simulink model "test_model_2018a1"  (R2018a)
settings: Solver=VariableStepAuto  StartTime=0.0  StopTime=4  RelTol=1e-3
values from neighbouring files (symbols this model uses):
  A = sys_d.A    [discreteTest.m]    (also in discreteTestAttacked.m)
  B = sys_d.B    [discreteTest.m]    (also in discreteTestAttacked.m)
  C = sys_d.C    [discreteTest.m]    (also in discreteTestAttacked.m)
  delta = steeringAngle(i)*(pi/180)*steering_ratio    [discreteTest.m]    (also in discreteTestAttacked.m)
  K = [   5.261, -0.023 ... (first row only)    [discreteTest.m]    (also in discreteTestAttacked.m)
  Ts = 0.04    [discreteTest.m]    (also in discreteTestAttacked.m)
undefined symbols (not defined in the file or in its folder): canChannel, L
libraries: canlib x6, canmsglib x4
settings Model: Creator=Shreyash  LastModifiedBy=Shreyash
settings SolverCC: AlgebraicLoopSolver=LineSearch

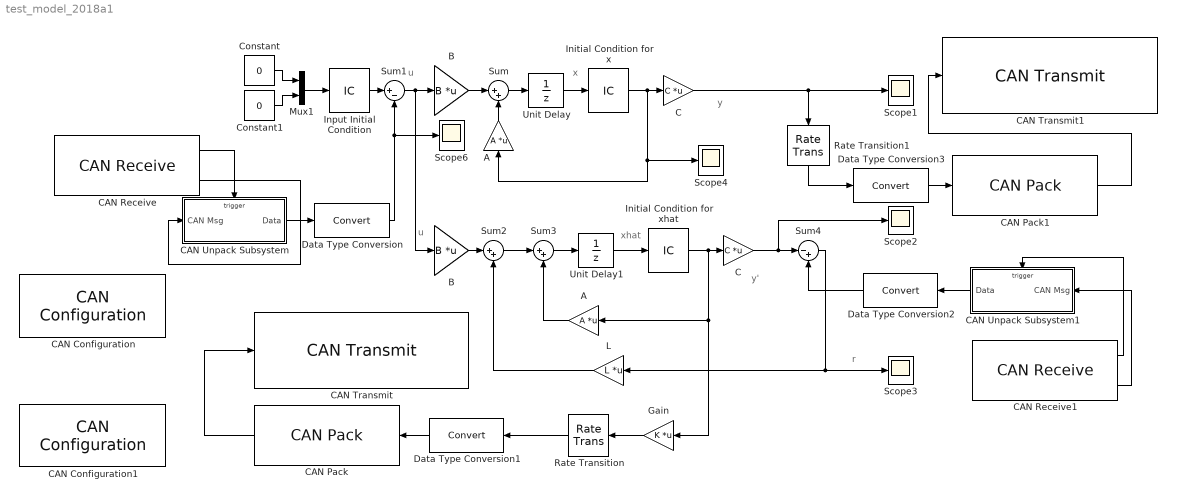
== system test_model_2018a1 ==
  note: y
  note: r
  note: y'
  note: u
  note: u
  note: x
  note: xhat
  A : Gain  Gain=A  Multiplication=Matrix(K*u)
  "A " : Gain  Gain=A  Multiplication=Matrix(K*u)
  B : Gain  Gain=B  Multiplication=Matrix(K*u)
  "B " : Gain  Gain=B  Multiplication=Matrix(K*u)
  C : Gain  Gain=C  Multiplication=Matrix(K*u)
  "C " : Gain  Gain=C  Multiplication=Matrix(K*u)
  CAN Configuration : canlib/CAN Configuration  BlockHandle=11.0004  DeviceMenu=MathWorks Virtual 1 (Channel 1)  Device=MathWorks Virtual 1 (Channel 1)  ObjConstructor=canChannel('MathWorks', 'Virtual 1', 1)  BusSpeed=500000  EnableBitParameters=off  AckMode=Normal
      settings: SourceProductName=Vehicle Network Toolbox  SourceProductBaseCode=VN
  CAN Configuration1 : canlib/CAN Configuration  BlockHandle=12.0004  DeviceMenu=MathWorks Virtual 1 (Channel 2)  Device=MathWorks Virtual 1 (Channel 2)  ObjConstructor=canChannel('MathWorks', 'Virtual 1', 2)  BusSpeed=500000  EnableBitParameters=off  AckMode=Normal
      settings: SourceProductName=Vehicle Network Toolbox  SourceProductBaseCode=VN
  CAN Pack : canmsglib/CAN Pack  MsgList=(none)  MsgName=CAN Msg  MsgIDType=Standard (11-bit identifier)  MsgIdentifier=500  MsgLength=8  NSignals=0  StartBits=0  SignalSizes=0  ByteOrders=0  DataTypes=0  MultiplexTypes=0  MultiplexValues=0  Factors=0  Offsets=0  Minimums=0  Maximums=0  Remote=off  ApplyMinMax=off  BusOutput=off
      settings: SourceProductName=Vehicle Network Toolbox  SourceProductBaseCode=VN  DataFormat=raw data
  CAN Pack1 : canmsglib/CAN Pack  MsgList=(none)  MsgName=CAN Msg  MsgIDType=Standard (11-bit identifier)  MsgIdentifier=500  MsgLength=8  NSignals=0  StartBits=0  SignalSizes=0  ByteOrders=0  DataTypes=0  MultiplexTypes=0  MultiplexValues=0  Factors=0  Offsets=0  Minimums=0  Maximums=0  Remote=off  ApplyMinMax=off  BusOutput=off
      settings: SourceProductName=Vehicle Network Toolbox  SourceProductBaseCode=VN  DataFormat=raw data
  CAN Receive : canlib/CAN Receive  BlockHandle=17.0004  DeviceMenu=MathWorks Virtual 1 (Channel 2)  Device=MathWorks Virtual 1 (Channel 2)  ObjConstructor=canChannel('MathWorks', 'Virtual 1', 2)  EnableStandardIDsFilter=off  StandardIDs=0  EnableExtendedIDsFilter=off  ExtendedIDs=0  SampleTime=0.04  MsgsPerTimestep=all  StdIDsCombo=Allow all  ExtIDsCombo=Allow all  InternalFilterUpdateStatus=on  BusOutput=off
      settings: SourceProductName=Vehicle Network Toolbox  SourceProductBaseCode=VN
  CAN Receive1 : canlib/CAN Receive  BlockHandle=18.0004  DeviceMenu=MathWorks Virtual 1 (Channel 2)  Device=MathWorks Virtual 1 (Channel 2)  ObjConstructor=canChannel('MathWorks', 'Virtual 1', 2)  EnableStandardIDsFilter=off  StandardIDs=0  EnableExtendedIDsFilter=off  ExtendedIDs=0  SampleTime=0.04  MsgsPerTimestep=all  StdIDsCombo=Allow all  ExtIDsCombo=Allow all  InternalFilterUpdateStatus=on  BusOutput=off
      settings: SourceProductName=Vehicle Network Toolbox  SourceProductBaseCode=VN
  CAN Transmit : canlib/CAN Transmit  BlockHandle=19.0004  DeviceMenu=MathWorks Virtual 1 (Channel 1)  Device=MathWorks Virtual 1 (Channel 1)  ObjConstructor=canChannel('MathWorks', 'Virtual 1', 1)  EnablePeriodicTransmit=on  MessagePeriod=0.04
      settings: SourceProductName=Vehicle Network Toolbox  SourceProductBaseCode=VN
  CAN Transmit1 : canlib/CAN Transmit  BlockHandle=20.0004  DeviceMenu=MathWorks Virtual 1 (Channel 1)  Device=MathWorks Virtual 1 (Channel 1)  ObjConstructor=canChannel('MathWorks', 'Virtual 1', 1)  EnablePeriodicTransmit=on  MessagePeriod=0.04
      settings: SourceProductName=Vehicle Network Toolbox  SourceProductBaseCode=VN
  CAN Unpack Subsystem : Subsystem  TreatAsAtomicUnit=on
  CAN Unpack Subsystem1 : Subsystem  TreatAsAtomicUnit=on
  Constant : Constant  Value=0
  Constant1 : Constant  Value=0
  Data Type Conversion : DataTypeConversion  SaturateOnIntegerOverflow=on
  Data Type Conversion1 : DataTypeConversion
  Data Type Conversion2 : DataTypeConversion  SaturateOnIntegerOverflow=on
  Data Type Conversion3 : DataTypeConversion
  Gain : Gain  Gain=K  Multiplication=Matrix(K*u)
  Initial Condition for x : InitialCondition  Value=[0.0005062279;0.0162158827]
  Initial Condition for xhat : InitialCondition  Value=[0;0]
  Input Initial Condition : InitialCondition  Value=[delta;0]
  L : Gain  Gain=L  Multiplication=Matrix(K*u)
  Mux1 : Mux  Inputs=2
  Rate Transition : RateTransition  Deterministic=off  InitialCondition=Ts  OutPortSampleTime=Ts
  Rate Transition1 : RateTransition  InitialCondition=Ts  OutPortSampleTime=Ts
  Scope{1..4,6} (5 alike) : Scope
  Sum : Sum  Inputs=|++
  Sum1 : Sum  Inputs=|+-
  Sum2 : Sum  Inputs=|++
  Sum3 : Sum  Inputs=|++
  Sum4 : Sum  Inputs=|-+
  Unit Delay : UnitDelay  SampleTime=-1
  Unit Delay1 : UnitDelay  SampleTime=-1
  wires:
  "B "/1 -> Sum/1
  Unit Delay/1 -> Initial Condition for x/1
  Sum/1 -> Unit Delay/1
  "A "/1 -> Sum/2
  Constant1/1 -> Mux1/2
  Constant/1 -> Mux1/1
  B/1 -> Sum2/1
  Sum2/1 -> Sum3/1
  Sum3/1 -> Unit Delay1/1
  Unit Delay1/1 -> Initial Condition for xhat/1
  L/1 -> Sum2/2
  A/1 -> Sum3/2
  Sum4/1 -> Scope3/1, L/1
  Initial Condition for x/1 -> Scope4/1, "A "/1, "C "/1
  C/1 -> Scope2/1, Sum4/1
  Initial Condition for xhat/1 -> A/1, Gain/1, C/1
  "C "/1 -> Rate Transition1/1, Scope1/1
  Sum1/1 -> B/1, "B "/1
  Mux1/1 -> Input Initial Condition/1
  Input Initial Condition/1 -> Sum1/1
  Gain/1 -> Rate Transition/1
  CAN Pack/1 -> CAN Transmit/1
  CAN Receive/2 -> CAN Unpack Subsystem/1(CAN Msg)
  CAN Unpack Subsystem/1(Data) -> Data Type Conversion/1
  Data Type Conversion/1 -> Scope6/1, Sum1/2
  CAN Receive/1 -> CAN Unpack Subsystem/Trigger
  Rate Transition/1 -> Data Type Conversion1/1
  Data Type Conversion1/1 -> CAN Pack/1
  Rate Transition1/1 -> Data Type Conversion3/1
  Data Type Conversion3/1 -> CAN Pack1/1
  CAN Pack1/1 -> CAN Transmit1/1
  Data Type Conversion2/1 -> Sum4/2
  CAN Unpack Subsystem1/1(Data) -> Data Type Conversion2/1
  CAN Receive1/2 -> CAN Unpack Subsystem1/1(CAN Msg)
  CAN Receive1/1 -> CAN Unpack Subsystem1/Trigger

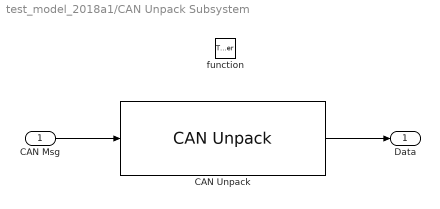
== system test_model_2018a1/CAN Unpack Subsystem ==
  CAN Msg : Inport
  function : TriggerPort  TriggerType=function-call  VariantControl=Variant
  CAN Unpack : canmsglib/CAN Unpack  MsgList=(none)  MsgName=CAN Msg  MsgIDType=Standard (11-bit identifier)  MsgIdentifier=500  MsgLength=1  NSignals=0  IDPort=off  TimestampPort=off  ErrorPort=off  RemotePort=off  LengthPort=off  StatusPort=off  StartBits=0  SignalSizes=0  ByteOrders=0  DataTypes=0  MultiplexTypes=0  MultiplexValues=0  Factors=0  Offsets=0  Minimums=0  Maximums=0  ApplyMinMax=off
      settings: SourceProductName=Vehicle Network Toolbox  SourceProductBaseCode=VN  DataFormat=raw data
  Data : Outport
  wires:
  CAN Msg/1 -> CAN Unpack/1
  CAN Unpack/1 -> Data/1

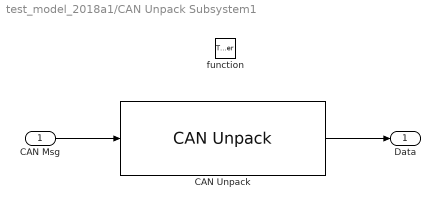
== system test_model_2018a1/CAN Unpack Subsystem1 ==
  CAN Msg : Inport
  function : TriggerPort  TriggerType=function-call  VariantControl=Variant
  CAN Unpack : canmsglib/CAN Unpack  MsgList=(none)  MsgName=CAN Msg  MsgIDType=Standard (11-bit identifier)  MsgIdentifier=500  MsgLength=1  NSignals=0  IDPort=off  TimestampPort=off  ErrorPort=off  RemotePort=off  LengthPort=off  StatusPort=off  StartBits=0  SignalSizes=0  ByteOrders=0  DataTypes=0  MultiplexTypes=0  MultiplexValues=0  Factors=0  Offsets=0  Minimums=0  Maximums=0  ApplyMinMax=off
      settings: SourceProductName=Vehicle Network Toolbox  SourceProductBaseCode=VN  DataFormat=raw data
  Data : Outport
  wires:
  CAN Msg/1 -> CAN Unpack/1
  CAN Unpack/1 -> Data/1
